simulink model "sysP1"  (R2023a)
settings: Solver=ode45  StartTime=0.0  StopTime=10  MaxStep=1E-3  RelTol=1e-3
libraries: slpidlib x1, simulink x1
settings Model: Creator=maria  LastModifiedBy=maria
settings DataIOCC: ReturnWorkspaceOutputs=off  TimeSaveName=t
settings DebuggingCC: AlgebraicLoopMsg=none  ArtificialAlgebraicLoopMsg=none  MaxConsecutiveZCsMsg=none  ModelReferenceExtraNoncontSigs=none  OperatingPointInterfaceChecksumMismatchMsg=none

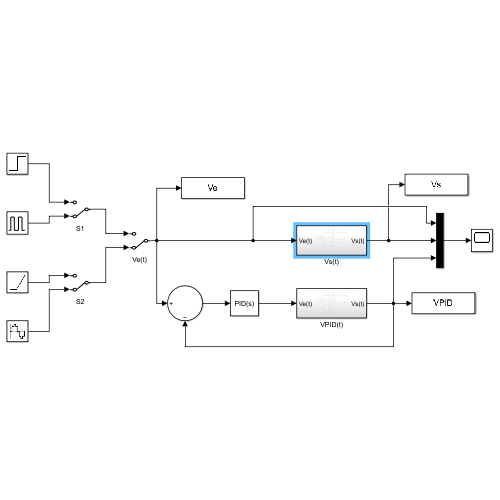
[thumbnail: Simulink's stored preview of the top-level diagram]
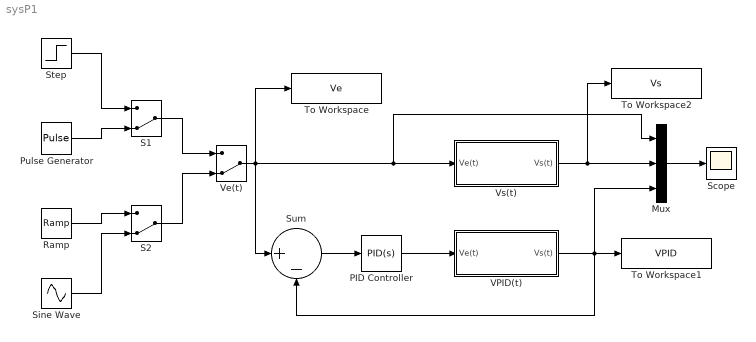
== system sysP1 ==
  Mux : Mux  Inputs=3
  PID Controller : slpidlib/PID Controller  Controller=PID  Form=Parallel  TimeDomain=Continuous-time  UseExternalTs=off  SampleTime=-1  IntegratorMethod=Forward Euler  FilterMethod=Forward Euler  ControllerParametersSource=internal  P=0.0869765982567339  I=782.855103427492  UseKiTs=off  D=0  N=100  UseFilter=on  TunerSelectOption=Transfer Function Based (PID Tuner App)  InitialConditionSource=internal  InitialConditionForIntegrator=0  InitialConditionForFilter=0  DifferentiatorICPrevScaledInput=0  ExternalReset=none  TrackingMode=off  Kt=1  LimitOutput=off  SatLimitsSource=internal  UpperSaturationLimit=inf  LowerSaturationLimit=-inf  LinearizeAsGain=on  AntiWindupMode=none  Kb=1  LimitIntegrator=off  UpperIntegratorSaturationLimit=inf  LowerIntegratorSaturationLimit=-inf  POutMin=[]  POutMax=[]  IOutMin=[]  IOutMax=[]  DOutMin=[]  DOutMax=[]  NOutMin=[]  NOutMax=[]  SumOutMin=[]  SumOutMax=[]  SaturationOutMin=[]  SaturationOutMax=[]  PParamMin=[]  PParamMax=[]  IParamMin=[]  IParamMax=[]  DParamMin=[]  DParamMax=[]  NParamMin=[]  NParamMax=[]  KbParamMin=[]  KbParamMax=[]  KtParamMin=[]  KtParamMax=[]  KbOutMin=[]  KbOutMax=[]  KtOutMin=[]  KtOutMax=[]  IntegratorOutMin=[]  IntegratorOutMax=[]  FilterOutMin=[]  FilterOutMax=[]  SumI1OutMin=[]  SumI1OutMax=[]  SumI2OutMin=[]  SumI2OutMax=[]  SumI3OutMin=[]  SumI3OutMax=[]  SumI4OutMin=[]  SumI4OutMax=[]  SumDOutMin=[]  SumDOutMax=[]  DifferentiatorOutMin=[]  DifferentiatorOutMax=[]  FilterDiffOutCoefMin=[]  FilterDiffOutCoefMax=[]  ReciprocalOutMin=[]  ReciprocalOutMax=[]  SumDenOutMin=[]  SumDenOutMax=[]  SumNumOutMin=[]  SumNumOutMax=[]  DivideOutMin=[]  DivideOutMax=[]  UdiffTsProdOutMin=[]  UdiffTsProdOutMax=[]  NTsProdOutMin=[]  NTsProdOutMax=[]  UintegralTsProdOutMin=[]  UintegralTsProdOutMax=[]  UngainTsProdOutMin=[]  UngainTsProdOutMax=[]  ClampingZeroOutDataTypeStr=Inherit: Inherit via back propagation  ClampingZeroOutMin=[]  ClampingZeroOutMax=[]  FilterDenConstantOutDataTypeStr=Inherit: Inherit via back propagation  FilterDenConstantOutMin=[]  FilterDenConstantOutMax=[]  PCopyOutDataTypeStr=Inherit: Inherit via back propagation  PCopyOutMin=[]  PCopyOutMax=[]  NCopyOutDataTypeStr=Inherit: Inherit via back propagation  NCopyOutMin=[]  NCopyOutMax=[]  IntegratorContinuousStateAttributes=''  IntegratorStateMustResolveToSignalObject=off  IntegratorRTWStateStorageClass=Auto  FilterContinuousStateAttributes=''  FilterStateMustResolveToSignalObject=off  FilterRTWStateStorageClass=Auto  ParallelPVariant=InternalParameters  IdealPVariant=Disabled  IVariant=InternalParameters  DVariant=InternalParameters  IntegratorVariant=Continuous  SatVariant=Disabled  AWVariant=Passthrough  PCopyVariant=Disabled  TRVariant=Disabled  FdbkBlocksVariant=Forward  IdealPFdbkVariant=Disabled  SatFdbkVariant=Disabled  DerivativeFilterVariant=ContFilter  NVariant=InternalParameters  NCopyVariant=Disabled  FilterICVariant=InternalICsFilter  IntegratorICVariant=InternalICs  ExternalResetVariant=Disabled  TRSumVariant=Passthrough  SumFdbkVariant=Disabled  SumVariant=Sum_PID  TsampFilterVariant=InternalTs  TsampNgainVariant=Passthrough  TsampIntegralVariant=Disabled_SignalSpec  ExternalSaturationOutDataTypeStr=Inherit: Same as second input
  Pulse Generator : DiscretePulseGenerator  PulseType=Time based  Period=10  PulseWidth=10  PhaseDelay=1
  Ramp : simulink/Sources/Ramp  slope=1/10  start=0  InitialOutput=0
  S1 : ManualSwitch  CurrentSetting=0
  S2 : ManualSwitch  CurrentSetting=0
  Scope : Scope
  Sine Wave : Sin  Frequency=1.5708  SampleTime=0.001
  Step : Step  Time=0
  Sum : Sum  Inputs=|+-
  To Workspace : ToWorkspace  VariableName=Ve  SampleTime=-1
  To Workspace1 : ToWorkspace  VariableName=VPID  SampleTime=-1
  To Workspace2 : ToWorkspace  VariableName=Vs  SampleTime=-1
  VPID(t) : Subsystem
  Ve(t) : ManualSwitch  CurrentSetting=0
  Vs(t) : Subsystem
  wires:
  Mux/1 -> Scope/1
  S1/1 -> Ve(t)/1
  S2/1 -> Ve(t)/2
  Step/1 -> S1/1
  Pulse Generator/1 -> S1/2
  Ramp/1 -> S2/1
  Sine Wave/1 -> S2/2
  PID Controller/1 -> VPID(t)/1(Ve(t))
  Sum/1 -> PID Controller/1
  Vs(t)/1(Vs(t)) -> Mux/2, To Workspace2/1
  VPID(t)/1(Vs(t)) -> Mux/3, Sum/2, To Workspace1/1
  Ve(t)/1 -> To Workspace/1, Sum/1, Mux/1, Vs(t)/1(Ve(t))

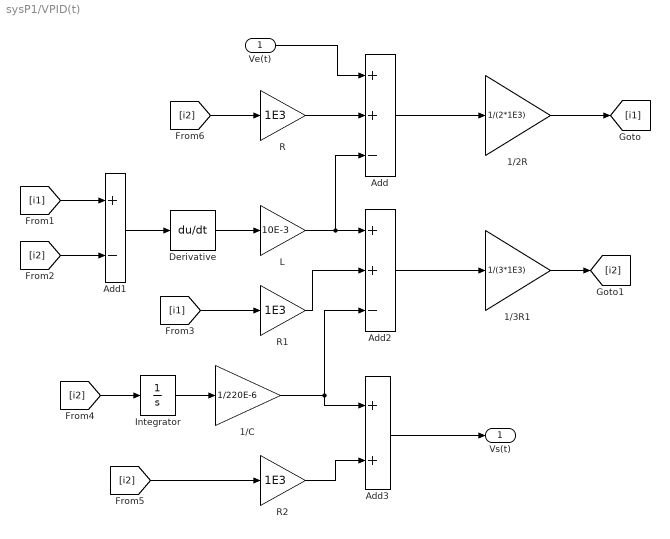
== system sysP1/VPID(t) ==
  Ve(t) : Inport
  1/2R : Gain  Gain=1/(2*1E3)
  1/3R1 : Gain  Gain=1/(3*1E3)
  1/C : Gain  Gain=1/220E-6
  Add : Sum  Inputs=++-
  Add1 : Sum  Inputs=+-
  Add2 : Sum  Inputs=++-
  Add3 : Sum
  Derivative : Derivative
  Integrator : Integrator
  L : Gain  Gain=10E-3
  R : Gain  Gain=1E3
  R1 : Gain  Gain=1E3
  R2 : Gain  Gain=1E3
  Vs(t) : Outport
  wires:
  Integrator/1 -> 1/C/1
  [i2] -> R2/1
  [i1] -> R1/1
  R1/1 -> Add2/2
  [i2] -> Integrator/1
  [i2] -> Add1/2
  R/1 -> Add/2
  Derivative/1 -> L/1
  Add/1 -> 1/2R/1
  [i1] -> Add1/1
  Add2/1 -> 1/3R1/1
  1/3R1/1 -> [i2]
  R2/1 -> Add3/2
  Add1/1 -> Derivative/1
  Ve(t)/1 -> Add/1
  1/2R/1 -> [i1]
  [i2] -> R/1
  L/1 -> Add2/1, Add/3
  1/C/1 -> Add3/1, Add2/3
  Add3/1 -> Vs(t)/1

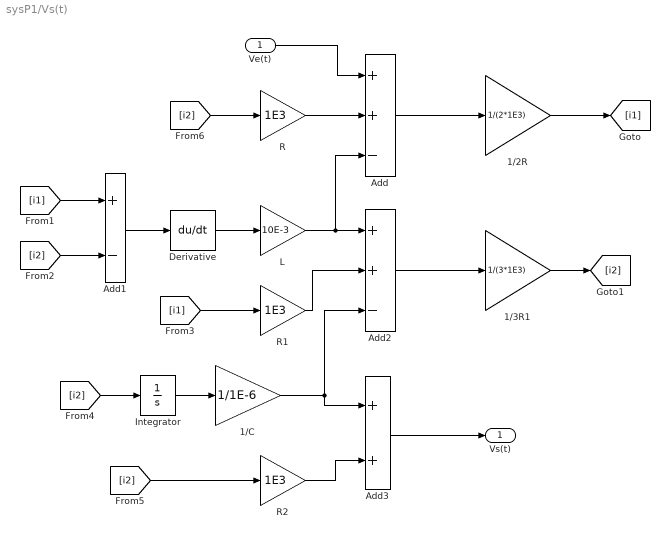
== system sysP1/Vs(t) ==
  Ve(t) : Inport
  1/2R : Gain  Gain=1/(2*1E3)
  1/3R1 : Gain  Gain=1/(3*1E3)
  1/C : Gain  Gain=1/1E-6
  Add : Sum  Inputs=++-
  Add1 : Sum  Inputs=+-
  Add2 : Sum  Inputs=++-
  Add3 : Sum
  Derivative : Derivative
  Integrator : Integrator
  L : Gain  Gain=10E-3
  R : Gain  Gain=1E3
  R1 : Gain  Gain=1E3
  R2 : Gain  Gain=1E3
  Vs(t) : Outport
  wires:
  Integrator/1 -> 1/C/1
  [i2] -> R2/1
  [i1] -> R1/1
  R1/1 -> Add2/2
  [i2] -> Integrator/1
  [i2] -> Add1/2
  R/1 -> Add/2
  Derivative/1 -> L/1
  Add/1 -> 1/2R/1
  [i1] -> Add1/1
  Add2/1 -> 1/3R1/1
  1/3R1/1 -> [i2]
  R2/1 -> Add3/2
  Add1/1 -> Derivative/1
  Ve(t)/1 -> Add/1
  1/2R/1 -> [i1]
  [i2] -> R/1
  L/1 -> Add2/1, Add/3
  1/C/1 -> Add3/1, Add2/3
  Add3/1 -> Vs(t)/1
